simulink model "iterative_motion_controller"  (R2025a)
settings: Solver=FixedStepDiscrete  StartTime=0.0  StopTime=1  RelTol=1e-3
undefined symbols (not defined in the file): AmcfocInitConf, MAX_EVENTS_PER_TICK, N_MOTORS, Ts_ControlFOC
settings Model: DataDictionary=amcfoc.sldd  Creator=mfussi  LastModifiedBy=mfussi
settings SolverCC: ConcurrentTasks=on  AutoInsertRateTranBlk=on  InsertRTBMode=Never (minimum delay)
settings DataIOCC: SaveOutput=off  SignalLogging=off  DSMLogging=off  SaveTime=off
settings OptimizationCC: DefaultParameterBehavior=Inlined  GainParamInheritBuiltInType=on  UseFloatMulNetSlope=on  DefaultUnderspecifiedDataType=single  UseSpecifiedMinMax=on  InlineInvariantSignals=on  PassReuseOutputArgsAs=Individual arguments  ZeroExternalMemoryAtStartup=off  ZeroInternalMemoryAtStartup=off  SimCompilerOptimization=on  OptimizeBlockOrder=speed  DifferentSizesBufferReuse=on  EfficientTunableParamExpr=on
settings DebuggingCC: ParameterTunabilityLossMsg=error
settings HardwareCC: ProdBitPerPointer=32.0  ProdBitPerSizeT=32.0  ProdBitPerPtrDiffT=32.0  ProdLargestAtomicInteger=Long  ProdLargestAtomicFloat=Double  ProdWordSize=32.0  ProdHWDeviceType=ARM Compatible->ARM Cortex-M
settings ModelReferenceCC: UpdateModelReferenceTargets=IfOutOfDate  EnableRefExpFcnMdlSchedulingChecks=on  ModelReferenceNumInstancesAllowed=Single
settings SFSimCC: MATLABDynamicMemAlloc=off
settings RTWCC: SystemTargetFile=ert.tlc  GenCodeOnly=on  PackageGeneratedCodeAndArtifacts=on  TemplateMakefile=ert_default_tmf  GenerateReport=on  RTWUseSimCustomCode=on  BuildConfiguration=Faster Runs  LaunchReport=on  TargetLang=C++  GenerateCodeMetricsReport=on  GenerateCodeReplacementReport=on  GPUComputeCapability=3.5  Description=Embedded Coder
settings CodeAppCC: ForceParamTrailComments=on  IgnoreCustomStorageClasses=off  MaxIdLength=60.0  OperatorAnnotations=on  SimulinkDataObjDesc=on  SFDataObjDesc=on  InsertBlockDesc=on
settings ERTTargetCC: ExtModeTransport=0.0  ExtModeStaticAlloc=off  ExtModeMexFile=ext_comm  ExtModeIntrfLevel=Level1  RootIOFormat=Structure reference  ERTCustomFileTemplate=example_file_process.tlc  DynamicArrayContainerType=coder::array  TargetLangStandard=C++03 (ISO)  CodeReplacementLibrary=iCubTech  CombineSignalStateStructs=on  SuppressErrorStatus=on  SupportNonFinite=off

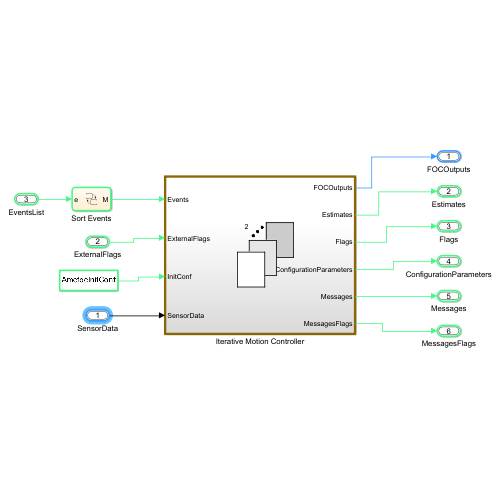
[thumbnail: Simulink's stored preview of the top-level diagram]
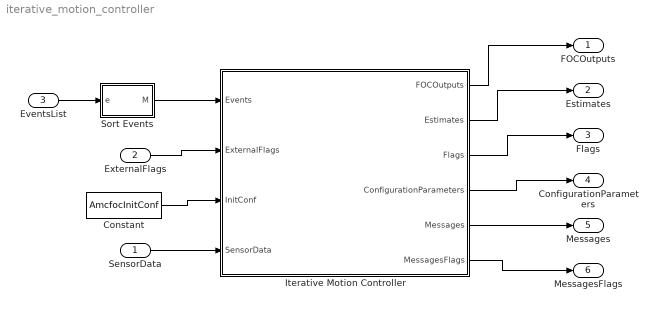
== system iterative_motion_controller ==
  SensorData : Inport  OutDataTypeStr=Bus: SensorsData  PortDimensions=N_MOTORS  SampleTime=Ts_ControlFOC  BusOutputAsStruct=on
  ExternalFlags : Inport  Port=2  OutDataTypeStr=Bus: ExternalFlags  BusOutputAsStruct=on
  EventsList : Inport  Port=3  OutDataTypeStr=Bus: ReceivedEvents  PortDimensions=N_MOTORS*MAX_EVENTS_PER_TICK  BusOutputAsStruct=on
  Constant : Constant  Value=AmcfocInitConf  OutDataTypeStr=Bus: ActuatorConfiguration  SampleTime=1e-3
  Iterative Motion Controller : Subsystem  TreatAsAtomicUnit=on
  Sort Events : Stateflow chart  TreatAsAtomicUnit=on
  FOCOutputs : Outport  OutDataTypeStr=Bus: FOCOutputs  BusOutputAsStruct=on
  Estimates : Outport  Port=2  OutDataTypeStr=Bus: EstimatedData  BusOutputAsStruct=on
  Flags : Outport  Port=3  OutDataTypeStr=Bus: Flags  BusOutputAsStruct=on
  ConfigurationParameters : Outport  Port=4  OutDataTypeStr=Bus: ActuatorConfiguration  BusOutputAsStruct=on
  Messages : Outport  Port=5  OutDataTypeStr=Bus: BUS_MESSAGES_TX  BusOutputAsStruct=on
  MessagesFlags : Outport  Port=6  OutDataTypeStr=Bus: BUS_STATUS_TX  BusOutputAsStruct=on
  wires:
  EventsList/1 -> Sort Events/1(e)
  ExternalFlags/1 -> Iterative Motion Controller/2(ExternalFlags)
  Sort Events/1(M) -> Iterative Motion Controller/1(Events)
  SensorData/1 -> Iterative Motion Controller/4(SensorData)
  Constant/1 -> Iterative Motion Controller/3(InitConf)
  Iterative Motion Controller/1(FOCOutputs) -> FOCOutputs/1
  Iterative Motion Controller/5(Messages) -> Messages/1
  Iterative Motion Controller/3(Flags) -> Flags/1
  Iterative Motion Controller/2(Estimates) -> Estimates/1
  Iterative Motion Controller/4(ConfigurationParameters) -> ConfigurationParameters/1
  Iterative Motion Controller/6(MessagesFlags) -> MessagesFlags/1

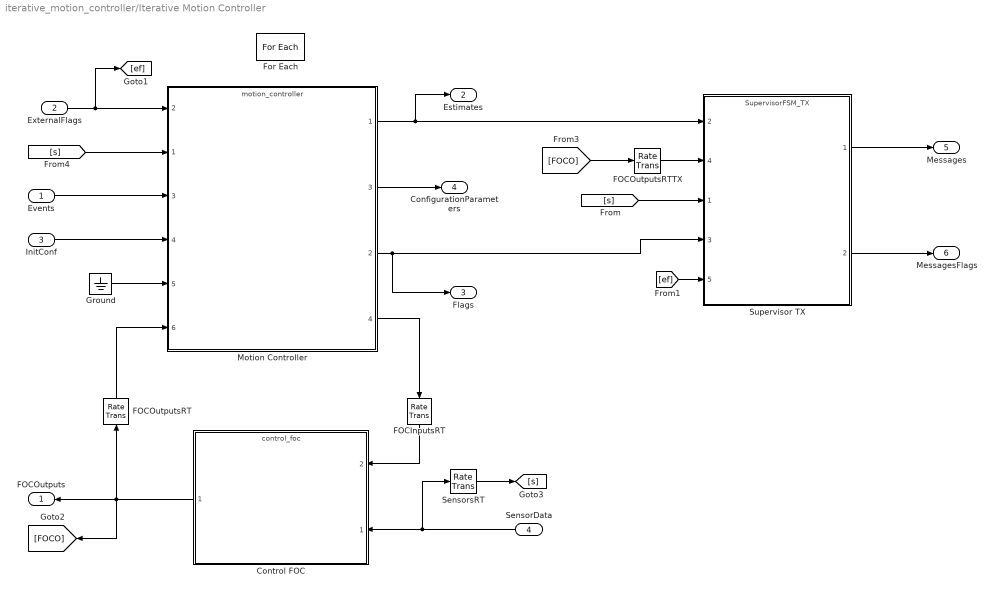
== system iterative_motion_controller/Iterative Motion Controller ==
  Events : Inport  OutDataTypeStr=Bus:ReceivedEvents  Partition=on  PartitionDimension=1  PartitionWidth=1  PartitionOffset=0
  ExternalFlags : Inport  Port=2  OutDataTypeStr=Bus: ExternalFlags
  InitConf : Inport  Port=3  OutDataTypeStr=Bus: ActuatorConfiguration  Partition=on  PartitionDimension=1  PartitionWidth=1  PartitionOffset=0
  SensorData : Inport  Port=4  OutDataTypeStr=Bus: SensorsData  SampleTime=Ts_ControlFOC  Partition=on  PartitionDimension=1  PartitionWidth=1  PartitionOffset=0
  Control FOC : ModelReference  ModelNameDialog=control_foc.slx  ModelReferenceVersion=9.5
      settings: PortSchema="{\"entries\":[{\"content\":{\"sides\":[{\"content\":{\"connectorIds\":[\"Out1\"]},\"type\":\"ConnectorPlacement.EquallySpacedRectSide\",\"uuid\":\"3d3ecbe0-23c4-4052-9ff0-e5eb2127c57e\"},{\"content\":{\"connectorIds\":[\"In2\",\"In1\"],\"side\":\"RIGHT\"},\"type\":\"ConnectorPlacement.EquallySpacedRectSide\",\"uuid\":\"40226699-f109-4440-bdec-f5fa54985f5e\"},{\"content\":{\"side\":\"TOP\"},\"type\":\"ConnectorPlacement.EquallySpacedRectSide\",\"uuid\":\"96b5eff6-eed9-43f4-aa86-2e804815aaee\"}]},\"type\":\"ConnectorPlacement.EquallySpacedConnector\",\"uuid\":\"74b92ba9-5721-4892-a04c-a2dba486add5\"}],\"packageUris\":[\"http://schema.mathworks.com/mf0/Connector/R2020b\"],\"version\":\"1.0\"}"
  FOCInputsRT : RateTransition  Deterministic=off  OutPortSampleTimeOpt=Inherit
  FOCOutputsRT : RateTransition  Deterministic=off  OutPortSampleTimeOpt=Inherit
  FOCOutputsRTTX : RateTransition  Deterministic=off  OutPortSampleTimeOpt=Inherit
  For Each : ForEach  DisableCoverage=on
  Ground : Ground
  Motion Controller : ModelReference  ModelNameDialog=motion_controller.slx  ModelReferenceVersion=5.36
      settings: PortSchema="{\"entries\":[{\"content\":{\"sides\":[{\"content\":{\"connectorIds\":[\"In2\",\"In1\",\"In3\",\"In4\",\"In5\",\"In6\"]},\"type\":\"ConnectorPlacement.EquallySpacedRectSide\",\"uuid\":\"379a1b60-57a2-4ccb-a061-d06c9ad096ee\"},{\"content\":{\"connectorIds\":[\"Out1\",\"Out3\",\"Out2\",\"Out4\"],\"side\":\"RIGHT\"},\"type\":\"ConnectorPlacement.EquallySpacedRectSide\",\"uuid\":\"27b3d028-7796-406c-a973-a0b783b604b2\"},{\"content\":{\"side\":\"TOP\"},\"type\":\"ConnectorPlacement.EquallySpacedRectSide\",\"uuid\":\"38e048f9-e5c6-4a39-8bca-9fbf31731ae5\"}]},\"type\":\"ConnectorPlacement.EquallySpacedConnector\",\"uuid\":\"97b4f620-742c-4215-a432-9dc15dd496c6\"}],\"packageUris\":[\"http://schema.mathworks.com/mf0/Connector/R2020b\"],\"version\":\"1.0\"}"
  "SensorsRT " : RateTransition  Deterministic=off  OutPortSampleTimeOpt=Inherit
  Supervisor TX : ModelReference  ModelNameDialog=SupervisorFSM_TX.slx  ModelReferenceVersion=10.25
      settings: PortSchema="{\"entries\":[{\"content\":{\"sides\":[{\"content\":{\"connectorIds\":[\"In2\",\"In4\",\"In1\",\"In3\",\"In5\"]},\"type\":\"ConnectorPlacement.EquallySpacedRectSide\",\"uuid\":\"da3a0c31-d41a-44f2-85ec-d1033079ee97\"},{\"content\":{\"connectorIds\":[\"Out1\",\"Out2\"],\"side\":\"RIGHT\"},\"type\":\"ConnectorPlacement.EquallySpacedRectSide\",\"uuid\":\"20109ca7-306f-4d99-aef0-3fab938882d1\"},{\"content\":{\"side\":\"TOP\"},\"type\":\"ConnectorPlacement.EquallySpacedRectSide\",\"uuid\":\"7be952f9-d28b-4eac-8fc6-f95f374eaa80\"}]},\"type\":\"ConnectorPlacement.EquallySpacedConnector\",\"uuid\":\"a950c446-ce16-41c8-9269-d83d512a5505\"}],\"packageUris\":[\"http://schema.mathworks.com/mf0/Connector/R2020b\"],\"version\":\"1.0\"}"
  FOCOutputs : Outport  OutDataTypeStr=Bus: FOCOutputs  ConcatenationDimension=1
  Estimates : Outport  Port=2  OutDataTypeStr=Bus: EstimatedData  ConcatenationDimension=1
  Flags : Outport  Port=3  OutDataTypeStr=Bus: Flags  ConcatenationDimension=1
  ConfigurationParameters : Outport  Port=4  OutDataTypeStr=Bus: ActuatorConfiguration  ConcatenationDimension=1
  Messages : Outport  Port=5  ConcatenationDimension=1
  MessagesFlags : Outport  Port=6  ConcatenationDimension=1
  wires:
  ExternalFlags/1 -> Motion Controller/2, [ef]
  InitConf/1 -> Motion Controller/4
  Events/1 -> Motion Controller/3
  [ef] -> Supervisor TX/5
  Supervisor TX/1 -> Messages/1
  Supervisor TX/2 -> MessagesFlags/1
  Ground/1 -> Motion Controller/5
  Motion Controller/1 -> Estimates/1, Supervisor TX/2
  Motion Controller/2 -> Flags/1, Supervisor TX/3
  Motion Controller/3 -> ConfigurationParameters/1
  Control FOC/1 -> [FOCO], FOCOutputsRT/1, FOCOutputs/1
  Motion Controller/4 -> FOCInputsRT/1
  SensorData/1 -> Control FOC/1, "SensorsRT "/1
  [FOCO] -> FOCOutputsRTTX/1
  [s] -> Motion Controller/1
  [s] -> Supervisor TX/1
  FOCOutputsRTTX/1 -> Supervisor TX/4
  "SensorsRT "/1 -> [s]
  FOCInputsRT/1 -> Control FOC/2
  FOCOutputsRT/1 -> Motion Controller/6

== stateflow chart iterative_motion_controller/Sort Events ==
  settings: initializeOutput=1
  (default) -> (junction 13) : % Bin Events
  (junction 13) -> (junction 15) : {idx = 0;
      | counter_motor_1 = 0;
      | counter_motor_2 = 0;}
  (junction 15) -> (junction 14) [order 1] : [idx < N_MOTORS*MAX_EVENTS_PER_TICK]
  (junction 14) -> (junction 60) [order 1] : [e[idx].motor_id == 0 && counter_motor_1 < MAX_EVENTS_PER_TICK]{
      | M[e[idx].motor_id][counter_motor_1] = e[idx];
      | counter_motor_1++;}
  (junction 14) -> (junction 61) [order 2] : [e[idx].motor_id == 1 && counter_motor_2 < MAX_EVENTS_PER_TICK]{
      | M[e[idx].motor_id][counter_motor_2 ] = e[idx];
      | counter_motor_2++;}
  (junction 17) -> (junction 15) : {idx++;}
  (junction 14) -> (junction 17) [order 3]
  (junction 60) -> (junction 61)
  (junction 15) -> (junction 59) [order 2]
  (junction 61) -> (junction 17)
  data: e input Bus: ReceivedEvents size=[N_MOTORS*MAX_EVENTS_PER_TICK]; M output Bus: ReceivedEvents size=[N_MOTORS, MAX_EVENTS_PER_TICK]; idx local uint8 size=1; counter_motor_1 local uint8 size=1; counter_motor_2 local uint8 size=1; MAX_EVENTS_PER_TICK parameter; N_MOTORS parameter
